simulink model "Gearbox"  (R2019b)
settings: Solver=VariableStepAuto  StartTime=0.0  StopTime=10.0  RelTol=1e-3
PreLoadFcn:
  | modelDir = fileparts(get_param(bdroot, 'FileName'));
  | addpath(fullfile(modelDir,'../../Parameters'));
  | 
  | Parameters_Model
  | Parameters_Simulation
  | Parameters_Controller
InitFcn:
  | Parameters_Model
  | Parameters_Simulation
  | Parameters_Controller
undefined symbols (not defined in the file): Bg, n
settings Model: Creator=Thomas  LastModifiedBy=thomas.jespersen
settings DataIOCC: ReturnWorkspaceOutputs=off
settings DebuggingCC: ArithmeticOperatorsInVariantConditions=warning
settings SFSimCC: SimUseLocalCustomCode=off  CustomCodeUndefinedFunction=UseInterfaceOnly
settings RTWCC: RTWUseLocalCustomCode=off

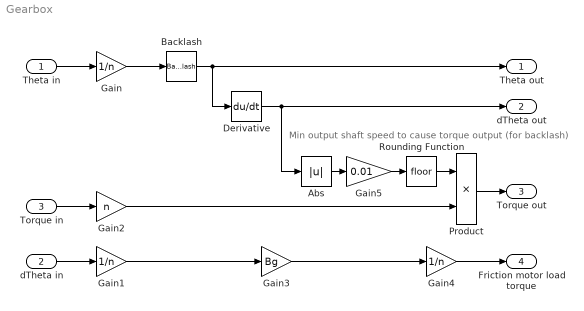
== system Gearbox ==
  note: Min output shaft speed to cause torque output (for backlash)
  Theta in : Inport
  dTheta in : Inport  Port=2
  Torque in : Inport  Port=3
  Abs : Abs
  Backlash : Backlash  BacklashWidth=theta_backlash
  Derivative : Derivative  CoefficientInTFapproximation=0.00001
  Gain : Gain  Gain=1/n
  Gain1 : Gain  Gain=1/n
  Gain2 : Gain  Gain=n
  Gain3 : Gain  Gain=Bg
  Gain4 : Gain  Gain=1/n
  Gain5 : Gain  Gain=0.01
  Product : Product
  Rounding Function : Rounding
  Theta out : Outport  VectorParamsAs1DForOutWhenUnconnected=off
  dTheta out : Outport  Port=2  VectorParamsAs1DForOutWhenUnconnected=off
  Torque out : Outport  Port=3  VectorParamsAs1DForOutWhenUnconnected=off
  Friction motor load torque : Outport  Port=4  VectorParamsAs1DForOutWhenUnconnected=off
  wires:
  Backlash/1 -> Derivative/1, Theta out/1
  Torque in/1 -> Gain2/1
  Gain2/1 -> Product/2
  Gain3/1 -> Gain4/1
  Gain4/1 -> Friction motor load torque/1
  dTheta in/1 -> Gain1/1
  Theta in/1 -> Gain/1
  Gain/1 -> Backlash/1
  Derivative/1 -> Abs/1, dTheta out/1
  Gain1/1 -> Gain3/1
  Abs/1 -> Gain5/1
  Gain5/1 -> Rounding Function/1
  Rounding Function/1 -> Product/1
  Product/1 -> Torque out/1
